simulink library "RI_MK"  (R2013b)
settings: Solver=ode45  StartTime=0.0  StopTime=10.0  RelTol=1e-3
libraries: RI_MK x1
settings Model: Creator=Szalay  LastModifiedBy=Szalay

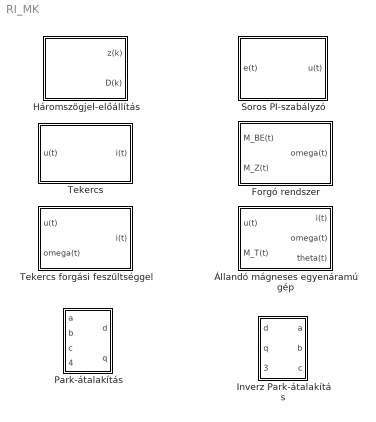
== system RI_MK ==
  Forgó rendszer : Subsystem  mask(Forgó rendszer){J=1, B=1e-3, omega_0=0}
      mask prompts: J "Tehetetlenségi nyomaték"; B "Forgási súrlódási együttható"; omega_0 "Kezdeti szögsebesség"
      mask help: Súrlódó tengely körül forgó test.
  Háromszögjel-előállítás : Subsystem  mask(Háromszögjel-előállítás){T_S=50e-3, A=2, f=1}
      mask prompts: T_S "Mintavételi idő"; A "Amplitúdó"; f "Frekvencia (Hz)"
      mask init:
      | N = round(1/(4*T_S*f));
  Inverz Park-átalakítás : Subsystem
  Park-átalakítás : Subsystem
  Soros PI-szabályzó : Subsystem  mask(Soros PI-szabályzó){K_PI=1, T_I=1}
      mask prompts: K_PI "Arányos tényező"; T_I "Integrálási időállandó"
      mask help: Egyszerű soros felépítésű PI-szabályzó.
      mask Display:
      | % Csatlakozók
      | port_label('input', 1, '{\ite}({\itt})', 'texmode', 'on');
      | port_label('output', 1, '{\itu}({\itt})', 'texmode', 'on');
      | 
      | % Felirat
      | text( ...
      |     0.5, 0.5, '{\bfPI_S}', ...
      |     'HorizontalAlignment', 'center', ...
      |     'texmode', 'on' ...
      |     );
  Tekercs : Subsystem  mask(Tekercs){R=1, L=1e-3, i_0=0}
      mask prompts: R "Ellenállás"; L "Öninduktivitás"; i_0 "Kezdeti áramerősség"
      mask help: Tekercs zavarás nélkül.
  Tekercs forgási feszültséggel : Subsystem  mask(Tekercs forgási feszültséggel){R=1, L=1e-3, Psi_0=1e-3, i_0=0, theta_0=0}
      mask prompts: R "Ellenállás"; L "Öninduktivitás"; Psi_0 "Az állandó mágnes tekercsfluxusa"; i_0 "Kezdeti áramerősség"; theta_0 "Kezdeti szöghelyzet"
      mask help: Tekercs zavarással.
  Állandó mágneses egyenáramú gép : Subsystem  mask(Állandó mágneses egyenáramú gép){R=1.76, L=658e-6, k_T=68.3e-3, k_E=68.3e-3, J=99.5e-7, B=5.7301e-06, i_0=0, omega_0=0, theta_0=0}
      mask prompts: R "Armatúra ellenállás"; L "Armatúra induktivitás"; k_T "Nyomatékállandó"; k_E "Feszültségállandó"; J "Tehetetlenségi nyomaték"; B "Forgási súrlódási együttható"; i_0 "Kezdeti áramerősség"; omega_0 "Kezdeti szögsebesség"; theta_0 "Kezdeti szöghelyzet"
      mask help:
      | <p>Az állandó mágneses egyenáramú gép modellje a
      | <b>Maxon DCX 35L</b> 48 V névleges feszültségű változata
      | alapján paraméterezve.</p>
      mask DialogControl Container5 Prompt: Kezdeti értékek
      mask Display:
      | % Csatlakozók
      | port_label('input', 1, '{\itu}({\itt})', 'texmode', 'on');
      | port_label('input', 2, '{\itM_T}({\itt})', 'texmode', 'on');
      | 
      | port_label('output', 1, '{\iti}({\itt})', 'texmode', 'on');
      | port_label('output', 2, '{\it\omega}({\itt})', 'texmode', 'on');
      | port_label('output', 3, '{\it\vartheta}({\itt})', 'texmode', 'on');
      | 
      | % Felirat
      | text(0.5, 0.5, '{\bfÁMEG}', 'HorizontalAlignment', 'center', 'texmode', 'on');

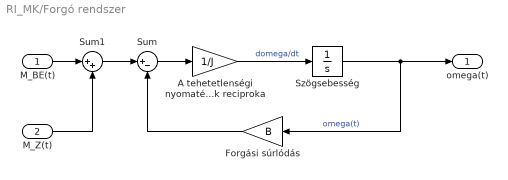
== system RI_MK/Forgó rendszer ==
  M_BE(t) : Inport
  M_Z(t) : Inport  Port=2
  A tehetetlenségi nyomaték reciproka : Gain  Gain=1/J
  Forgási súrlódás : Gain  Gain=B
  Sum : Sum  Inputs=|+-
  Sum1 : Sum  Inputs=|++
  Szögsebesség : Integrator  InitialCondition=omega_0
  omega(t) : Outport
  wires:
  Szögsebesség/1 -> omega(t)/1, Forgási súrlódás/1  "omega(t)"
  Sum/1 -> A tehetetlenségi nyomaték reciproka/1
  A tehetetlenségi nyomaték reciproka/1 -> Szögsebesség/1  "domega/dt"
  Forgási súrlódás/1 -> Sum/2
  M_BE(t)/1 -> Sum1/1
  Sum1/1 -> Sum/1
  M_Z(t)/1 -> Sum1/2

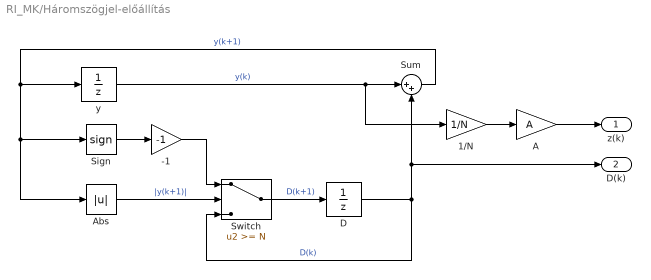
== system RI_MK/Háromszögjel-előállítás ==
  -1 : Gain  Gain=-1
  1/N : Gain  Gain=1/N
  A : Gain  Gain=A
  Abs : Abs
  D : UnitDelay  InitialCondition=-1  SampleTime=T_S
  Sign : Signum
  Sum : Sum  Inputs=|++
  Switch : Switch  Threshold=N
  y : UnitDelay  InitialCondition=N  SampleTime=T_S
  z(k) : Outport
  D(k) : Outport  Port=2
  wires:
  -1/1 -> Switch/1
  Sum/1 -> Abs/1, Sign/1, y/1  "y(k+1)"
  Switch/1 -> D/1  "D(k+1)"
  y/1 -> Sum/1, 1/N/1  "y(k)"
  Sign/1 -> -1/1
  D/1 -> Switch/3, Sum/2, D(k)/1  "D(k)"
  Abs/1 -> Switch/2  "|y(k+1)|"
  1/N/1 -> A/1
  A/1 -> z(k)/1

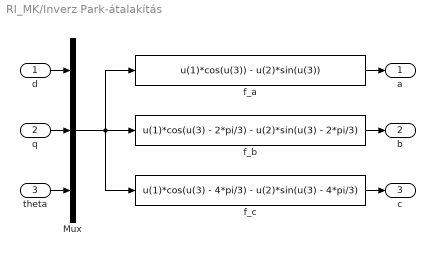
== system RI_MK/Inverz Park-átalakítás ==
  d : Inport
  q : Inport  Port=2
  theta : Inport  Port=3
  Mux : Mux  Inputs=3
  f_a : Fcn  Expr=u(1)*cos(u(3)) - u(2)*sin(u(3))
  f_b : Fcn  Expr=u(1)*cos(u(3) - 2*pi/3) - u(2)*sin(u(3) - 2*pi/3)
  f_c : Fcn  Expr=u(1)*cos(u(3) - 4*pi/3) - u(2)*sin(u(3) - 4*pi/3)
  a : Outport
  b : Outport  Port=2
  c : Outport  Port=3
  wires:
  d/1 -> Mux/1
  f_c/1 -> c/1
  f_b/1 -> b/1
  f_a/1 -> a/1
  theta/1 -> Mux/3
  q/1 -> Mux/2
  Mux/1 -> f_c/1, f_b/1, f_a/1

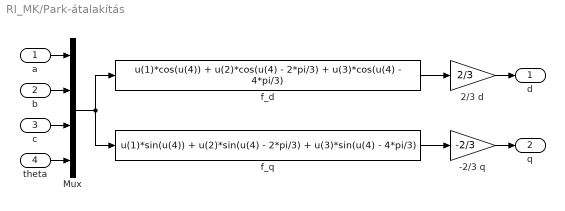
== system RI_MK/Park-átalakítás ==
  a : Inport
  b : Inport  Port=2
  c : Inport  Port=3
  theta : Inport  Port=4
  -2/3 q : Gain  Gain=-2/3
  2/3 d : Gain  Gain=2/3
  Mux : Mux
  f_d : Fcn  Expr=u(1)*cos(u(4)) + u(2)*cos(u(4) - 2*pi/3) + u(3)*cos(u(4) - 4*pi/3)
  f_q : Fcn  Expr=u(1)*sin(u(4)) + u(2)*sin(u(4) - 2*pi/3) + u(3)*sin(u(4) - 4*pi/3)
  d : Outport
  q : Outport  Port=2
  wires:
  f_d/1 -> 2/3 d/1
  Mux/1 -> f_d/1, f_q/1
  f_q/1 -> -2/3 q/1
  theta/1 -> Mux/4
  a/1 -> Mux/1
  2/3 d/1 -> d/1
  b/1 -> Mux/2
  c/1 -> Mux/3
  -2/3 q/1 -> q/1

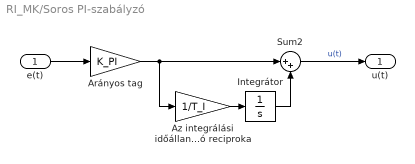
== system RI_MK/Soros PI-szabályzó ==
  e(t) : Inport
  Arányos tag : Gain  Gain=K_PI
  Az integrálási időállandó reciproka : Gain  Gain=1/T_I
  Integrátor : Integrator
  Sum2 : Sum  Inputs=|++
  u(t) : Outport
  wires:
  Arányos tag/1 -> Sum2/1, Az integrálási időállandó reciproka/1
  Integrátor/1 -> Sum2/2
  Az integrálási időállandó reciproka/1 -> Integrátor/1
  Sum2/1 -> u(t)/1  "u(t)"
  e(t)/1 -> Arányos tag/1

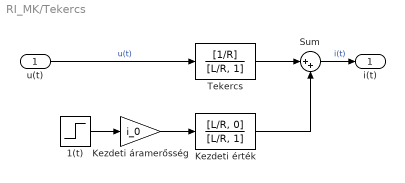
== system RI_MK/Tekercs ==
  u(t) : Inport
  1(t) : Step  Time=0  SampleTime=0
  Kezdeti áramerősség : Gain  Gain=i_0
  Kezdeti érték : TransferFcn  Numerator=[L/R, 0]  Denominator=[L/R, 1]
  Sum : Sum  Inputs=|++
  Tekercs : TransferFcn  Numerator=[1/R]  Denominator=[L/R, 1]
  i(t) : Outport
  wires:
  u(t)/1 -> Tekercs/1  "u(t)"
  Tekercs/1 -> Sum/1
  1(t)/1 -> Kezdeti áramerősség/1
  Kezdeti áramerősség/1 -> Kezdeti érték/1
  Sum/1 -> i(t)/1  "i(t)"
  Kezdeti érték/1 -> Sum/2

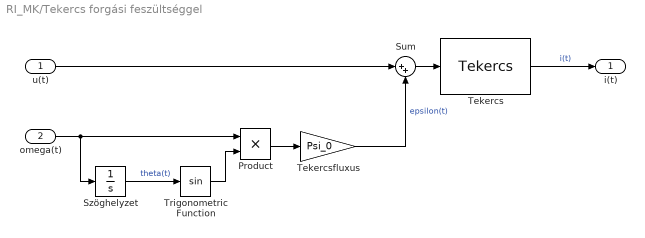
== system RI_MK/Tekercs forgási feszültséggel ==
  u(t) : Inport
  omega(t) : Inport  Port=2
  Product : Product
  Sum : Sum  Inputs=|++
  Szöghelyzet : Integrator  InitialCondition=theta_0
  Tekercs : RI_MK/Tekercs  R=R  L=L  i_0=i_0
  Tekercsfluxus : Gain  Gain=Psi_0
  Trigonometric Function : Trigonometry
  i(t) : Outport
  wires:
  u(t)/1 -> Sum/1
  Product/1 -> Tekercsfluxus/1
  Tekercsfluxus/1 -> Sum/2  "epsilon(t)"
  Trigonometric Function/1 -> Product/2
  Szöghelyzet/1 -> Trigonometric Function/1  "theta(t)"
  omega(t)/1 -> Product/1, Szöghelyzet/1
  Tekercs/1 -> i(t)/1  "i(t)"
  Sum/1 -> Tekercs/1

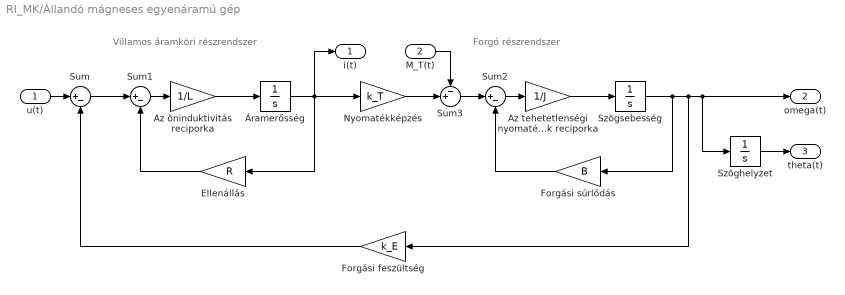
== system RI_MK/Állandó mágneses egyenáramú gép ==
  note: Villamos áramköri részrendszer
  note: Forgó részrendszer
  u(t) : Inport
  M_T(t) : Inport  Port=2
  Az tehetetlenségi nyomaték reciporka : Gain  Gain=1/J
  Az öninduktivitás reciporka : Gain  Gain=1/L
  Ellenállás : Gain  Gain=R
  Forgási feszültség : Gain  Gain=k_E
  Forgási súrlódás : Gain  Gain=B
  Nyomatékképzés : Gain  Gain=k_T
  Sum : Sum  Inputs=|+-
  Sum1 : Sum  Inputs=|+-
  Sum2 : Sum  Inputs=|+-
  Sum3 : Sum  Inputs=-+|
  Szöghelyzet : Integrator  InitialCondition=theta_0
  Szögsebesség : Integrator  InitialCondition=omega_0
  Áramerősség : Integrator  InitialCondition=i_0
  i(t) : Outport
  omega(t) : Outport  Port=2
  theta(t) : Outport  Port=3
  wires:
  u(t)/1 -> Sum/1
  Sum1/1 -> Az öninduktivitás reciporka/1
  Ellenállás/1 -> Sum1/2
  Az öninduktivitás reciporka/1 -> Áramerősség/1
  Áramerősség/1 -> Nyomatékképzés/1, i(t)/1, Ellenállás/1
  Sum2/1 -> Az tehetetlenségi nyomaték reciporka/1
  Forgási súrlódás/1 -> Sum2/2
  Az tehetetlenségi nyomaték reciporka/1 -> Szögsebesség/1
  Szögsebesség/1 -> Forgási feszültség/1, Szöghelyzet/1, omega(t)/1, Forgási súrlódás/1
  Nyomatékképzés/1 -> Sum3/2
  M_T(t)/1 -> Sum3/1
  Sum3/1 -> Sum2/1
  Sum/1 -> Sum1/1
  Forgási feszültség/1 -> Sum/2
  Szöghelyzet/1 -> theta(t)/1
